simulink model "FIR_Filter"  (R2019b)
settings: Solver=FixedStepAuto  StartTime=0.0  StopTime=10.0  FixedStep=0.2  RelTol=1e-3
model workspace (MAT data in the model file):
  a0 = 1
  a1 = 2
  a2 = -3
  a3 = -4
  a4 = 5
settings Model: Creator=Shreyas  LastModifiedBy=Shreyas
settings DataIOCC: SaveOutput=off  SaveTime=off

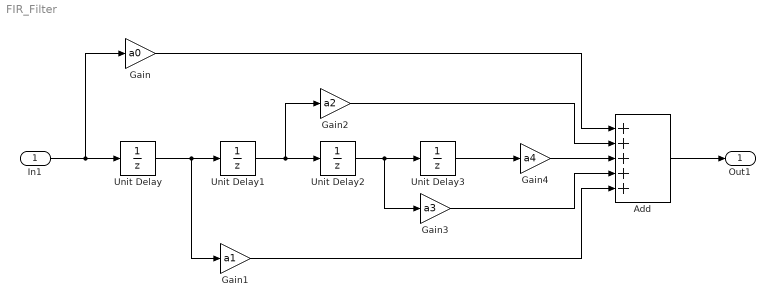
== system FIR_Filter ==
  In1 : Inport  OutDataTypeStr=double  PortDimensions=1  SampleTime=[0.20000000000000001,0]
  Add : Sum  Inputs=+++++
  Gain : Gain  Gain=a0
  Gain1 : Gain  Gain=a1
  Gain2 : Gain  Gain=a2
  Gain3 : Gain  Gain=a3
  Gain4 : Gain  Gain=a4
  Unit Delay{,1..3} (4 alike) : UnitDelay  SampleTime=-1  HasFrameUpgradeWarning=on
  Out1 : Outport  OutDataTypeStr=double  PortDimensions=1  SampleTime=[0.20000000000000001,0]
  wires:
  Unit Delay2/1 -> Unit Delay3/1, Gain3/1
  Gain/1 -> Add/1
  Unit Delay3/1 -> Gain4/1
  In1/1 -> Unit Delay/1, Gain/1
  Gain3/1 -> Add/4
  Gain4/1 -> Add/3
  Gain1/1 -> Add/5
  Unit Delay/1 -> Unit Delay1/1, Gain1/1
  Gain2/1 -> Add/2
  Unit Delay1/1 -> Unit Delay2/1, Gain2/1
  Add/1 -> Out1/1
